simulink model "regulator3"  (R2025b)
settings: Solver=VariableStepAuto  StartTime=0.0  StopTime=20  RelTol=1e-3
values from neighbouring files (symbols this model uses):
  D = 10    [zadanie4.m]
  I = 15    [zadanie4.m]    (also in zadanie5.m = 0)
  P = 100    [zadanie4.m]    (also in zadanie5.m = 2)
settings Model: Creator=micha  LastModifiedBy=Michał

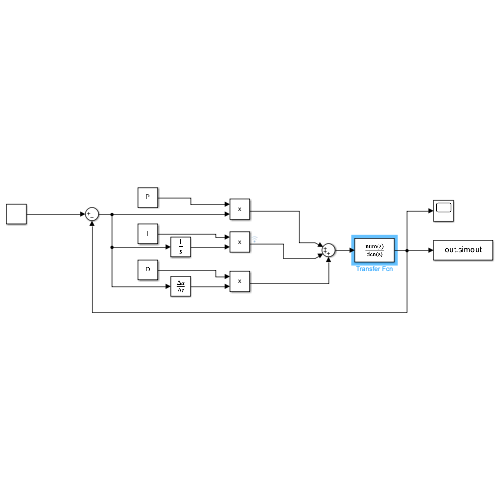
[thumbnail: Simulink's stored preview of the top-level diagram]
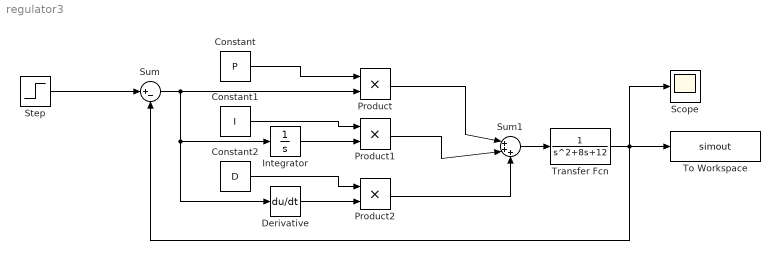
== system regulator3 ==
  Constant : Constant  Value=P
  Constant1 : Constant  Value=I  SampleTime=0
  Constant2 : Constant  Value=D
  Derivative : Derivative
  Integrator : Integrator
  Product : Product
  Product1 : Product
  Product2 : Product
  Scope : Scope
      settings: SampleTime=0.0001  ActiveDisplayYMinimum=-0.015243902439021576  ActiveDisplayYMaximum=0.13719512195119421
  Step : Step  SampleTime=0
  Sum : Sum  Inputs=|+-
  Sum1 : Sum  Inputs=|+++
  To Workspace : ToWorkspace  VariableName=simout  SaveFormat=Timeseries  SampleTime=-1
  Transfer Fcn : TransferFcn  Numerator=1  Denominator=[1 8 12]
  wires:
  Step/1 -> Sum/1
  Sum/1 -> Derivative/1, Integrator/1, Product/2
  Transfer Fcn/1 -> Sum/2, Scope/1, To Workspace/1
  Sum1/1 -> Transfer Fcn/1
  Constant/1 -> Product/1
  Product/1 -> Sum1/1
  Derivative/1 -> Product2/2
  Integrator/1 -> Product1/2
  Product2/1 -> Sum1/3
  Product1/1 -> Sum1/2
  Constant1/1 -> Product1/1
  Constant2/1 -> Product2/1
